simulink model "SingleTrackCANoe"  (R2021b)
settings: Solver=ode1  StartTime=0  StopTime=2  FixedStep=1.0000000000000000e-003  RelTol=1e-3
InitFcn:
  | sampleTime = str2double(get_param(bdroot, 'FixedStep'));
undefined symbols (not defined in the file or in its folder): AccPedalPos, BrakePedalPos, BrakeSwitch, DiscIntNeverNeededParam, DYNA4, EngSpd, IgnitionSwitch, InitialGear, InitialSpeed, IntendedEngTrq, LeftIndicator, MainBrakePress, MaxGear, MDL, MinGear, RefAcc, RefLane, RefLatPos, RefPath, RefPathCurv, RefSpd, RefSpdPreview, RefSpdRetrospect, RightIndicator, SteeringWheelAng, SteeringWheelTrq, UserDefinedRefValue, vm_const
libraries: UtilitiesLibrary x62, simulink x18, WheelSystemModules x14, LongitudinalControllerModules x13, LateralControllerModules x7, AnimationBusselectorModules x5, EnvironmentModules x5, BasicEngineControlModules x5, MiscellaneousControlModules x5, Animation3Modules x4, AuxiliariesModules x4, ReducedTireModules x4
(part 16 of 34)

== system SingleTrackCANoe/SimulationModel/Vehicle/WheelSystem/WheelSystemOutputs ==
  FrontLeftInnerTireStates : Inport
  FrontLeftTireStates : Inport  Port=2
  FrontLeftWheelStates : Inport  Port=3
  FrontRightInnerTireStates : Inport  Port=4
  FrontRightTireStates : Inport  Port=5
  FrontRightWheelStates : Inport  Port=6
  RearLeftInnerTireStates : Inport  Port=7
  RearLeftTireStates : Inport  Port=8
  RearLeftWheelStates : Inport  Port=9
  RearRightInnerTireStates : Inport  Port=10
  RearRightTireStates : Inport  Port=11
  RearRightWheelStates : Inport  Port=12
  FrontLeftOuput : Subsystem  Tag=TESIS DYNAware Interface Block  mask{NeedsUpdate=off, SignalInfo=|}
      mask SignalInfo=|
      | {
      |   "Version": "4.6",
      |   "MuxedOutputBusName": "FrontLeft",
      |   "MuxedInputBusName": "input",
      |   "MuxedInputSelected": false,
      |   "MuxedOutputSelected": true,
      |   "SignalData": [
      |     {
      |       "initialValue": "0.0",
      |       "name": "InnerTire",
      |       "comment": "",
      |       "minString": "",
      |       "maxString": "",
      |       "width": -1,
      |       "dataType": 0,
      |       "signalType": 1,
      |       "createSignal": false,
      |       "outputName": "InnerTire",
      |       "generateSignalAccessBlock": false,
      |       "accessId": "$(parentId).$(blockName).$(outputName)"
      |     },
      |     {
      |       "initialValue": "0.0",
      |       "name": "Tire",
      |       "comment": "",
      |       "minString": "",
      |       "maxString": "",
      |       "width": -1,
      |       "dataType": 0,
      |       "signalType": 1,
      |       "createSignal": false,
      |       "outputName": "Tire",
      |       "generateSignalAccessBlock": false,
      |       "accessId": "$(parentId).$(blockName).$(outputName)"
      |     },
      |     {
      |       "initialValue": "0.0",
      |       "name": "Wheel",
      |       "comment": "",
      |       "minString": "",
      |       "maxString": "",
      |       "width": -1,
      |       "dataType": 0,
      |       "signalType": 1,
      |       "createSignal": false,
      |       "outputName": "Wheel",
      |       "generateSignalAccessBlock": false,
      |       "accessId": "$(parentId).$(blockName).$(outputName)"
      |     }
      |   ]
      | }
      mask prompts: NeedsUpdate "Specify, if subsystem content needs to be updated"; SignalInfo "Signal Info (json)"
      mask help: DYNA4 Interface Block Version 4.6
      mask init:
      | blockName = get_param(gcbh, 'Name');
      | parentId = DYNA4.ModelHandling.AccessID.getFromHierarchy(gcbh);
      | TD.InterfaceBlock.ModelCallbacks.GenerateContent(gcb);
      settings: DeleteFcn=TD.InterfaceBlock.ModelCallbacks.CloseGUI( gcbh );  NameChangeFcn=TD.InterfaceBlock.ModelCallbacks.BlockRenamedHandler(gcbh);  OpenFcn=TD.InterfaceBlock.ModelCallbacks.OpenGUI( gcbh );  CloseFcn=TD.InterfaceBlock.ModelCallbacks.CloseGUI( gcbh );
      mask Display:
      | image('InterfaceBlock.png','center');
      | port_label('input',1, 'InnerTire');
      | port_label('input',2, 'Tire');
      | port_label('input',3, 'Wheel');
      | port_label('output',1, 'FrontLeft');
  FrontRightOuput : Subsystem  Tag=TESIS DYNAware Interface Block  mask{NeedsUpdate=off, SignalInfo=|}
      mask SignalInfo=|
      | {
      |   "Version": "4.6",
      |   "MuxedOutputBusName": "FrontRight",
      |   "MuxedInputBusName": "input",
      |   "MuxedInputSelected": false,
      |   "MuxedOutputSelected": true,
      |   "SignalData": [
      |     {
      |       "initialValue": "0.0",
      |       "name": "InnerTire",
      |       "comment": "",
      |       "minString": "",
      |       "maxString": "",
      |       "width": -1,
      |       "dataType": 0,
      |       "signalType": 1,
      |       "createSignal": false,
      |       "outputName": "InnerTire",
      |       "generateSignalAccessBlock": false,
      |       "accessId": "$(parentId).$(blockName).$(outputName)"
      |     },
      |     {
      |       "initialValue": "0.0",
      |       "name": "Tire",
      |       "comment": "",
      |       "minString": "",
      |       "maxString": "",
      |       "width": -1,
      |       "dataType": 0,
      |       "signalType": 1,
      |       "createSignal": false,
      |       "outputName": "Tire",
      |       "generateSignalAccessBlock": false,
      |       "accessId": "$(parentId).$(blockName).$(outputName)"
      |     },
      |     {
      |       "initialValue": "0.0",
      |       "name": "Wheel",
      |       "comment": "",
      |       "minString": "",
      |       "maxString": "",
      |       "width": -1,
      |       "dataType": 0,
      |       "signalType": 1,
      |       "createSignal": false,
      |       "outputName": "Wheel",
      |       "generateSignalAccessBlock": false,
      |       "accessId": "$(parentId).$(blockName).$(outputName)"
      |     }
      |   ]
      | }
      mask prompts: NeedsUpdate "Specify, if subsystem content needs to be updated"; SignalInfo "Signal Info (json)"
      mask help: DYNA4 Interface Block Version 4.6
      mask init:
      | blockName = get_param(gcbh, 'Name');
      | parentId = DYNA4.ModelHandling.AccessID.getFromHierarchy(gcbh);
      | TD.InterfaceBlock.ModelCallbacks.GenerateContent(gcb);
      settings: DeleteFcn=TD.InterfaceBlock.ModelCallbacks.CloseGUI( gcbh );  NameChangeFcn=TD.InterfaceBlock.ModelCallbacks.BlockRenamedHandler(gcbh);  OpenFcn=TD.InterfaceBlock.ModelCallbacks.OpenGUI( gcbh );  CloseFcn=TD.InterfaceBlock.ModelCallbacks.CloseGUI( gcbh );
      mask Display:
      | image('InterfaceBlock.png','center');
      | port_label('input',1, 'InnerTire');
      | port_label('input',2, 'Tire');
      | port_label('input',3, 'Wheel');
      | port_label('output',1, 'FrontRight');
  RearLeftOuput : Subsystem  Tag=TESIS DYNAware Interface Block  mask{NeedsUpdate=off, SignalInfo=|}
      mask SignalInfo=|
      | {
      |   "Version": "4.6",
      |   "MuxedOutputBusName": "RearLeft",
      |   "MuxedInputBusName": "input",
      |   "MuxedInputSelected": false,
      |   "MuxedOutputSelected": true,
      |   "SignalData": [
      |     {
      |       "initialValue": "0.0",
      |       "name": "InnerTire",
      |       "comment": "",
      |       "minString": "",
      |       "maxString": "",
      |       "width": -1,
      |       "dataType": 0,
      |       "signalType": 1,
      |       "createSignal": false,
      |       "outputName": "InnerTire",
      |       "generateSignalAccessBlock": false,
      |       "accessId": "$(parentId).$(blockName).$(outputName)"
      |     },
      |     {
      |       "initialValue": "0.0",
      |       "name": "Tire",
      |       "comment": "",
      |       "minString": "",
      |       "maxString": "",
      |       "width": -1,
      |       "dataType": 0,
      |       "signalType": 1,
      |       "createSignal": false,
      |       "outputName": "Tire",
      |       "generateSignalAccessBlock": false,
      |       "accessId": "$(parentId).$(blockName).$(outputName)"
      |     },
      |     {
      |       "initialValue": "0.0",
      |       "name": "Wheel",
      |       "comment": "",
      |       "minString": "",
      |       "maxString": "",
      |       "width": -1,
      |       "dataType": 0,
      |       "signalType": 1,
      |       "createSignal": false,
      |       "outputName": "Wheel",
      |       "generateSignalAccessBlock": false,
      |       "accessId": "$(parentId).$(blockName).$(outputName)"
      |     }
      |   ]
      | }
      mask prompts: NeedsUpdate "Specify, if subsystem content needs to be updated"; SignalInfo "Signal Info (json)"
      mask help: DYNA4 Interface Block Version 4.6
      mask init:
      | blockName = get_param(gcbh, 'Name');
      | parentId = DYNA4.ModelHandling.AccessID.getFromHierarchy(gcbh);
      | TD.InterfaceBlock.ModelCallbacks.GenerateContent(gcb);
      settings: DeleteFcn=TD.InterfaceBlock.ModelCallbacks.CloseGUI( gcbh );  NameChangeFcn=TD.InterfaceBlock.ModelCallbacks.BlockRenamedHandler(gcbh);  OpenFcn=TD.InterfaceBlock.ModelCallbacks.OpenGUI( gcbh );  CloseFcn=TD.InterfaceBlock.ModelCallbacks.CloseGUI( gcbh );
      mask Display:
      | image('InterfaceBlock.png','center');
      | port_label('input',1, 'InnerTire');
      | port_label('input',2, 'Tire');
      | port_label('input',3, 'Wheel');
      | port_label('output',1, 'RearLeft');
  RearRightOuput : Subsystem  Tag=TESIS DYNAware Interface Block  mask{NeedsUpdate=off, SignalInfo=|}
      mask SignalInfo=|
      | {
      |   "Version": "4.6",
      |   "MuxedOutputBusName": "RearRight",
      |   "MuxedInputBusName": "input",
      |   "MuxedInputSelected": false,
      |   "MuxedOutputSelected": true,
      |   "SignalData": [
      |     {
      |       "initialValue": "0.0",
      |       "name": "InnerTire",
      |       "comment": "",
      |       "minString": "",
      |       "maxString": "",
      |       "width": -1,
      |       "dataType": 0,
      |       "signalType": 1,
      |       "createSignal": false,
      |       "outputName": "InnerTire",
      |       "generateSignalAccessBlock": false,
      |       "accessId": "$(parentId).$(blockName).$(outputName)"
      |     },
      |     {
      |       "initialValue": "0.0",
      |       "name": "Tire",
      |       "comment": "",
      |       "minString": "",
      |       "maxString": "",
      |       "width": -1,
      |       "dataType": 0,
      |       "signalType": 1,
      |       "createSignal": false,
      |       "outputName": "Tire",
      |       "generateSignalAccessBlock": false,
      |       "accessId": "$(parentId).$(blockName).$(outputName)"
      |     },
      |     {
      |       "initialValue": "0.0",
      |       "name": "Wheel",
      |       "comment": "",
      |       "minString": "",
      |       "maxString": "",
      |       "width": -1,
      |       "dataType": 0,
      |       "signalType": 1,
      |       "createSignal": false,
      |       "outputName": "Wheel",
      |       "generateSignalAccessBlock": false,
      |       "accessId": "$(parentId).$(blockName).$(outputName)"
      |     }
      |   ]
      | }
      mask prompts: NeedsUpdate "Specify, if subsystem content needs to be updated"; SignalInfo "Signal Info (json)"
      mask help: DYNA4 Interface Block Version 4.6
      mask init:
      | blockName = get_param(gcbh, 'Name');
      | parentId = DYNA4.ModelHandling.AccessID.getFromHierarchy(gcbh);
      | TD.InterfaceBlock.ModelCallbacks.GenerateContent(gcb);
      settings: DeleteFcn=TD.InterfaceBlock.ModelCallbacks.CloseGUI( gcbh );  NameChangeFcn=TD.InterfaceBlock.ModelCallbacks.BlockRenamedHandler(gcbh);  OpenFcn=TD.InterfaceBlock.ModelCallbacks.OpenGUI( gcbh );  CloseFcn=TD.InterfaceBlock.ModelCallbacks.CloseGUI( gcbh );
      mask Display:
      | image('InterfaceBlock.png','center');
      | port_label('input',1, 'InnerTire');
      | port_label('input',2, 'Tire');
      | port_label('input',3, 'Wheel');
      | port_label('output',1, 'RearRight');
  WheelRear2_3Output : WheelSystemModules/WheelRear2_3Output  SystemSampleTime=-1  VariantActivationTime=update diagram  Latency=0  AutoFrameSizeCalculation=off
  WheelSystemOutput : Subsystem  Tag=TESIS DYNAware Interface Block  mask{NeedsUpdate=off, SignalInfo=|}
      mask SignalInfo=|
      | {
      |   "Version": "4.6",
      |   "MuxedOutputBusName": "WheelSystem",
      |   "MuxedInputBusName": "input",
      |   "MuxedInputSelected": false,
      |   "MuxedOutputSelected": true,
      |   "SignalData": [
      |     {
      |       "initialValue": "0.0",
      |       "name": "FrontLeft",
      |       "comment": "",
      |       "minString": "",
      |       "maxString": "",
      |       "width": -1,
      |       "dataType": 0,
      |       "signalType": 1,
      |       "createSignal": false,
      |       "outputName": "FrontLeft",
      |       "generateSignalAccessBlock": false,
      |       "accessId": "$(parentId).$(blockName).$(outputName)"
      |     },
      |     {
      |       "initialValue": "0.0",
      |       "name": "FrontRight",
      |       "comment": "",
      |       "minString": "",
      |       "maxString": "",
      |       "width": -1,
      |       "dataType": 0,
      |       "signalType": 1,
      |       "createSignal": false,
      |       "outputName": "FrontRight",
      |       "generateSignalAccessBlock": false,
      |       "accessId": "$(parentId).$(blockName).$(outputName)"
      |     },
      |     {
      |       "initialValue": "0.0",
      |       "name": "RearLeft",
      |       "comment": "",
      |       "minString": "",
      |       "maxString": "",
      |       "width": -1,
      |       "dataType": 0,
      |       "signalType": 1,
      |       "createSignal": false,
      |       "outputName": "RearLeft",
      |       "generateSignalAccessBlock": false,
      |       "accessId": "$(parentId).$(blockName).$(outputName)"
      |     },
      |     {
      |       "initialValue": "0.0",
      |       "name": "RearRight",
      |       "comment": "",
      |       "minString": "",
      |       "maxString": "",
      |       "width": -1,
      |       "dataType": 0,
      |       "signalType": 1,
      |       "createSignal": false,
      |       "outputName": "RearRight",
      |       "generateSignalAccessBlock": false,
      |       "accessId": "$(parentId).$(blockName).$(outputName)"
      |     },
      |     {
      |       "initialValue": "0.0",
      |       "name": "Rear2Left",
      |       "comment": "",
      |       "minString": "",
      |       "maxString": "",
      |       "width": -1,
      |       "dataType": 0,
      |       "signalType": 1,
      |       "createSignal": false,
      |       "outputName": "Rear2Left",
      |       "generateSignalAccessBlock": false,
      |       "accessId": "$(parentId).$(blockName).$(outputName)"
      |     },
      |     {
      |       "initialValue": "0.0",
      |       "name": "Rear2Right",
      |       "comment": "",
      |       "minString": "",
      |       "maxString": "",
      |       "width": -1,
      |       "dataType": 0,
      |       "signalType": 1,
      |       "createSignal": false,
      |       "outputName": "Rear2Right",
      |       "generateSignalAccessBlock": false,
      |       "accessId": "$(parentId).$(blockName).$(outputName)"
      |     },
      |     {
      |       "initialValue": "0.0",
      |       "name": "Rear3Left",
      |       "comment": "",
      |       "minString": "",
      |       "maxString": "",
      |       "width": -1,
      |       "dataType": 0,
      |       "signalType": 1,
      |       "createSignal": false,
      |       "outputName": "Rear3Left",
      |       "generateSignalAccessBlock": false,
      |       "accessId": "$(parentId).$(blockName).$(outputName)"
      |     },
      |     {
      |       "initialValue": "0.0",
      |       "name": "Rear3Right",
      |       "comment": "",
      |       "minString": "",
      |       "maxString": "",
      |       "width": -1,
      |       "dataType": 0,
      |       "signalType": 1,
      |       "createSignal": false,
      |       "outputName": "Rear3Right",
      |       "generateSignalAccessBlock": false,
      |       "accessId": "$(parentId).$(blockName).$(outputName)"
      |     }
      |   ]
      | }
      mask prompts: NeedsUpdate "Specify, if subsystem content needs to be updated"; SignalInfo "Signal Info (json)"
      mask help: DYNA4 Interface Block Version 4.6
      mask init:
      | blockName = get_param(gcbh, 'Name');
      | parentId = DYNA4.ModelHandling.AccessID.getFromHierarchy(gcbh);
      | TD.InterfaceBlock.ModelCallbacks.GenerateContent(gcb);
      settings: DeleteFcn=TD.InterfaceBlock.ModelCallbacks.CloseGUI( gcbh );  NameChangeFcn=TD.InterfaceBlock.ModelCallbacks.BlockRenamedHandler(gcbh);  OpenFcn=TD.InterfaceBlock.ModelCallbacks.OpenGUI( gcbh );  CloseFcn=TD.InterfaceBlock.ModelCallbacks.CloseGUI( gcbh );
      mask Display:
      | image('InterfaceBlock.png','center');
      | port_label('input',1, 'FrontLeft');
      | port_label('input',2, 'FrontRight');
      | port_label('input',3, 'RearLeft');
      | port_label('input',4, 'RearRight');
      | port_label('input',5, 'Rear2Left');
      | port_label('input',6, 'Rear2Right');
      | port_label('input',7, 'Rear3Left');
      | port_label('input',8, 'Rear3Right');
      | port_label('output',1, 'WheelSystem');
  WheelSystem : Outport  VectorParamsAs1DForOutWhenUnconnected=off
  wires:
  FrontLeftInnerTireStates/1 -> FrontLeftOuput/1(InnerTire___UNIQUE_1)
  FrontLeftTireStates/1 -> FrontLeftOuput/2(Tire___UNIQUE_1)
  FrontLeftWheelStates/1 -> FrontLeftOuput/3(Wheel___UNIQUE_1)
  RearLeftInnerTireStates/1 -> RearLeftOuput/1(InnerTire___UNIQUE_1)
  RearLeftTireStates/1 -> RearLeftOuput/2(Tire___UNIQUE_1)
  RearLeftWheelStates/1 -> RearLeftOuput/3(Wheel___UNIQUE_1)
  RearRightInnerTireStates/1 -> RearRightOuput/1(InnerTire___UNIQUE_1)
  RearRightTireStates/1 -> RearRightOuput/2(Tire___UNIQUE_1)
  RearRightWheelStates/1 -> RearRightOuput/3(Wheel___UNIQUE_1)
  FrontLeftOuput/1(FrontLeft___UNIQUE_1) -> WheelSystemOutput/1(FrontLeft___UNIQUE_1)
  FrontRightOuput/1(FrontRight___UNIQUE_1) -> WheelSystemOutput/2(FrontRight___UNIQUE_1)
  RearLeftOuput/1(RearLeft___UNIQUE_1) -> WheelSystemOutput/3(RearLeft___UNIQUE_1)
  RearRightOuput/1(RearRight___UNIQUE_1) -> WheelSystemOutput/4(RearRight___UNIQUE_1)
  WheelSystemOutput/1(WheelSystem___UNIQUE_1) -> WheelSystem/1
  FrontRightInnerTireStates/1 -> FrontRightOuput/1(InnerTire___UNIQUE_1)
  FrontRightTireStates/1 -> FrontRightOuput/2(Tire___UNIQUE_1)
  FrontRightWheelStates/1 -> FrontRightOuput/3(Wheel___UNIQUE_1)
  WheelRear2_3Output/1 -> WheelSystemOutput/5(Rear2Left___UNIQUE_1), WheelSystemOutput/6(Rear2Right___UNIQUE_1), WheelSystemOutput/7(Rear3Left___UNIQUE_1), WheelSystemOutput/8(Rear3Right___UNIQUE_1)

== system SingleTrackCANoe/SimulationModel/VehicleControl/InitialConditions/InitialConditionsOutput ==
  InitialPositionX(WorldSys)[m]___UNIQUE_1 : Inport  Description=|  PortDimensions=[1]
      | <name>InitialPositionX(WorldSys)[m]</name>
      | <comment>Initial x-position in world coordinates</comment>
  InitialPositionY(WorldSys)[m]___UNIQUE_1 : Inport  Description=|  Port=2  PortDimensions=[1]
      | <name>InitialPositionY(WorldSys)[m]</name>
      | <comment>Initial y-position in world coordinates</comment>
  InitialPositionZ(WorldSys)[m]___UNIQUE_1 : Inport  Description=|  Port=3  PortDimensions=[1]
      | <name>InitialPositionZ(WorldSys)[m]</name>
      | <comment>Initial z-position in world coordinates</comment>
  InitialRoll[rad]___UNIQUE_1 : Inport  Description=|  Port=4  PortDimensions=[1]
      | <name>InitialRoll[rad]</name>
      | <comment>Initial roll angle</comment>
  InitialPitch[rad]___UNIQUE_1 : Inport  Description=|  Port=5  PortDimensions=[1]
      | <name>InitialPitch[rad]</name>
      | <comment>Initial pitch angle</comment>
  InitialYaw[rad]___UNIQUE_1 : Inport  Description=|  Port=6  PortDimensions=[1]
      | <name>InitialYaw[rad]</name>
      | <comment>Initial yaw angle</comment>
  __TDD__InitialConditions.InitialPitch[rad] : Demux  Outputs=[1]
  __TDD__InitialConditions.InitialPositionX(WorldSys)[m] : Demux  Outputs=[1]
  __TDD__InitialConditions.InitialPositionY(WorldSys)[m] : Demux  Outputs=[1]
  __TDD__InitialConditions.InitialPositionZ(WorldSys)[m] : Demux  Outputs=[1]
  __TDD__InitialConditions.InitialRoll[rad] : Demux  Outputs=[1]
  __TDD__InitialConditions.InitialYaw[rad] : Demux  Outputs=[1]
  __TDO__InitialConditions : BusCreator  Inputs=6
  InitialConditions___UNIQUE_1 : Outport  Description=|  PortDimensions=[6]  VectorParamsAs1DForOutWhenUnconnected=off
      | <name>InitialPositionX(WorldSys)[m]</name>
      | <comment>Initial x-position in world coordinates</comment>
  wires:
  InitialPositionX(WorldSys)[m]___UNIQUE_1/1 -> __TDD__InitialConditions.InitialPositionX(WorldSys)[m]/1
  __TDD__InitialConditions.InitialPositionX(WorldSys)[m]/1 -> __TDO__InitialConditions/1  "InitialPositionX(WorldSys)[m]"
  InitialPositionY(WorldSys)[m]___UNIQUE_1/1 -> __TDD__InitialConditions.InitialPositionY(WorldSys)[m]/1
  __TDD__InitialConditions.InitialPositionY(WorldSys)[m]/1 -> __TDO__InitialConditions/2  "InitialPositionY(WorldSys)[m]"
  InitialPositionZ(WorldSys)[m]___UNIQUE_1/1 -> __TDD__InitialConditions.InitialPositionZ(WorldSys)[m]/1
  __TDD__InitialConditions.InitialPositionZ(WorldSys)[m]/1 -> __TDO__InitialConditions/3  "InitialPositionZ(WorldSys)[m]"
  InitialRoll[rad]___UNIQUE_1/1 -> __TDD__InitialConditions.InitialRoll[rad]/1
  __TDD__InitialConditions.InitialRoll[rad]/1 -> __TDO__InitialConditions/4  "InitialRoll[rad]"
  InitialPitch[rad]___UNIQUE_1/1 -> __TDD__InitialConditions.InitialPitch[rad]/1
  __TDD__InitialConditions.InitialPitch[rad]/1 -> __TDO__InitialConditions/5  "InitialPitch[rad]"
  InitialYaw[rad]___UNIQUE_1/1 -> __TDD__InitialConditions.InitialYaw[rad]/1
  __TDD__InitialConditions.InitialYaw[rad]/1 -> __TDO__InitialConditions/6  "InitialYaw[rad]"
  __TDO__InitialConditions/1 -> InitialConditions___UNIQUE_1/1  "InitialConditions"

== system SingleTrackCANoe/SimulationModel/VehicleControl/LateralControl/Disabled LateralControl ==
  SchedulerAbscissae : Inport
  CtrlSystemsAbscissae : Inport  Port=2
  PhaseTerminationVals : Inport  Port=3
  VehicleInfo : Inport  Port=4
  LatCTRL : Inport  Port=5
  ExtCtrlVariablesEnforced : Inport  Port=6
  ExtCtrlVals : Inport  Port=7
  ControlSystems : Subsystem
  ControlSystemsPreprocessor : Subsystem
  DynaSystemInfo : Subsystem  Tag=DynaSystemInfo
      mask init:
      | data = get_param(gcb, 'UserData');
      settings: OpenFcn=DYNA4.ModelHandling.System.ShowEditSystemInformationDialog(gcb);
      mask Display: disp(['Type = ', data.type, '\nName = ', data.name ])
  Terminator{,1..6} (7 alike) : Terminator
  LateralControl : Outport  VectorParamsAs1DForOutWhenUnconnected=off
  wires:
  CtrlSystemsAbscissae/1 -> Terminator6/1
  VehicleInfo/1 -> Terminator5/1
  SchedulerAbscissae/1 -> Terminator/1
  PhaseTerminationVals/1 -> Terminator1/1
  LatCTRL/1 -> Terminator4/1
  ExtCtrlVariablesEnforced/1 -> Terminator2/1
  ExtCtrlVals/1 -> Terminator3/1
  ControlSystems/1(LateralControl) -> LateralControl/1

== system SingleTrackCANoe/SimulationModel/VehicleControl/LateralControl/Enabled LateralControl ==
  SchedulerAbscissae : Inport
  CtrlSystemsAbscissae : Inport  Port=2
  PhaseTerminationVals : Inport  Port=3
  VehicleInfo : Inport  Port=4
  LatCTRL : Inport  Port=5
  ExtCtrlVariablesEnforced : Inport  Port=6
  ExtCtrlVals : Inport  Port=7
  ControlSystems : Subsystem
  ControlSystemsPreprocessor : Subsystem
  DynaSystemInfo : Subsystem  Tag=DynaSystemInfo
      mask init:
      | data = get_param(gcb, 'UserData');
      settings: OpenFcn=DYNA4.ModelHandling.System.ShowEditSystemInformationDialog(gcb);
      mask Display: disp(['Type = ', data.type, '\nName = ', data.name ])
  LateralControl : Outport  VectorParamsAs1DForOutWhenUnconnected=off
  wires:
  ControlSystems/1(LateralControl) -> LateralControl/1
  ExtCtrlVals/1 -> ControlSystemsPreprocessor/5(ExtCtrlVals)
  ExtCtrlVariablesEnforced/1 -> ControlSystemsPreprocessor/4(ExtCtrlVariablesEnforced)
  LatCTRL/1 -> ControlSystemsPreprocessor/3(LatCTRL)
  PhaseTerminationVals/1 -> ControlSystemsPreprocessor/2(PhaseTerminationVals)
  SchedulerAbscissae/1 -> ControlSystemsPreprocessor/1(SchedulerAbscissae)
  ControlSystemsPreprocessor/4(ControlInputs) -> ControlSystems/4(ControlInputs)
  ControlSystemsPreprocessor/3(SourceIdentifiers) -> ControlSystems/3(SourceIdentifiers)
  ControlSystemsPreprocessor/2(TaskIdentifiers) -> ControlSystems/2(TaskIdentifiers)
  VehicleInfo/1 -> ControlSystems/6(VehicleInfo), ControlSystemsPreprocessor/7(VehicleInfo)
  CtrlSystemsAbscissae/1 -> ControlSystems/7(CtrlSystemsAbscissae)
  ControlSystems/2(ControllerParameters) -> ControlSystemsPreprocessor/6(ControllerParameters)
  ControlSystemsPreprocessor/5(UserDefinedSignals) -> ControlSystems/5(UserDefinedSignals)
  ControlSystemsPreprocessor/1(Phase[-]) -> ControlSystems/1(Phase[-])

== system SingleTrackCANoe/SimulationModel/VehicleControl/LongitudinalControl/ControlSystems ==
  note: SpeedControl Params Module has to be located here,
      | because its PreviewTime parameter is used in other controllers, too.
  SimulationTime[s] : Inport
  Phase[-] : Inport  Port=2
  TaskIdentifiers : Inport  Port=3
  SourceIdentifiers : Inport  Port=4
  ControlInputs : Inport  Port=5
  VehicleInfoSpeedControl : Inport  Port=6
  UserDefinedSignals : Inport  Port=7
  CtrlSystemsAbscissae : Inport  Port=8
  Brake System Switch and Pedal Limitation : Subsystem
  CreateOutputBus : Subsystem
  DynaSystemInfo : Subsystem  Tag=DynaSystemInfo
      mask init:
      | data = get_param(gcb, 'UserData');
      settings: OpenFcn=DYNA4.ModelHandling.System.ShowEditSystemInformationDialog(gcb);
      mask Display: disp(['Type = ', data.type, '\nName = ', data.name ])
  Longitudinal Controller : Subsystem
  ShiftControl : LongitudinalControllerModules/ShiftControl  DATA_NODE=MDL.VehicleControl.LongitudinalControl.ControlSystems.ShiftControl  UpshiftScalingMap=MDL.VehicleControl.LongitudinalControl.ControlSystems.ShiftControl.ShiftingSpeeds.UpshiftScalingMap  DownshiftScalingMap=MDL.VehicleControl.LongitudinalControl.ControlSystems.ShiftControl.ShiftingSpeeds.DownshiftScalingMap  UpshiftOffsetMap=MDL.VehicleControl.LongitudinalControl.ControlSystems.ShiftControl.ShiftingSpeeds.UpshiftOffsetMap  DownshiftOffsetMap=MDL.VehicleControl.LongitudinalControl.ControlSystems.ShiftControl.ShiftingSpeeds.DownshiftOffsetMap  UpshiftAbsoluteSpdMap=MDL.VehicleControl.LongitudinalControl.ControlSystems.ShiftControl.ShiftingSpeeds.UpshiftAbsoluteSpdMap  DownshiftAbsoluteSpdMap=MDL.VehicleControl.LongitudinalControl.ControlSystems.ShiftControl.ShiftingSpeeds.DownshiftAbsoluteSpdMap  MinGearShiftTimeConst=MDL.VehicleControl.LongitudinalControl.ControlSystems.ShiftControl.ShiftingParameters.MinGearShiftTimeConst  NeutralToFirstGearScaling=MDL.VehicleControl.LongitudinalControl.ControlSystems.ShiftControl.ShiftingParameters.NeutralToFirstGearScaling  UpshiftAllowedWheelSlip=MDL.VehicleControl.LongitudinalControl.ControlSystems.ShiftControl.ShiftingParameters.UpshiftAllowedWheelSlip  DownshiftAllowedWheelSlip=MDL.VehicleControl.LongitudinalControl.ControlSystems.ShiftControl.ShiftingParameters.DownshiftAllowedWheelSlip  GearShiftDelayTime=MDL.VehicleControl.LongitudinalControl.ControlSystems.ShiftControl.ShiftingParameters.GearShiftDelayTime  ClutchEngageEngSpd=MDL.VehicleControl.LongitudinalControl.ControlSystems.ShiftControl.ClutchParameters.ClutchEngageEngSpd  ClutchDisengageEngSpd=MDL.VehicleControl.LongitudinalControl.ControlSystems.ShiftControl.ClutchParameters.ClutchDisengageEngSpd  ClutchDelayTime=MDL.VehicleControl.LongitudinalControl.ControlSystems.ShiftControl.ClutchParameters.ClutchDelayTime  ClutchOpenSlewRate=MDL.VehicleControl.LongitudinalControl.ControlSystems.ShiftControl.ClutchParameters.ClutchOpenSlewRate  ClutchCloseSlewRate=MDL.VehicleControl.LongitudinalControl.ControlSystems.ShiftControl.ClutchParameters.ClutchCloseSlewRate  ClutchOpeningTime=MDL.VehicleControl.LongitudinalControl.ControlSystems.ShiftControl.ClutchParameters.ClutchOpeningTime  AccPedalOpenSlewRate=MDL.VehicleControl.LongitudinalControl.ControlSystems.ShiftControl.AcceleratorPedalParameters.AccPedalOpenSlewRate  AccPedalCloseSlewRate=MDL.VehicleControl.LongitudinalControl.ControlSystems.ShiftControl.AcceleratorPedalParameters.AccPedalCloseSlewRate  ReducedAccPedalTime=MDL.VehicleControl.LongitudinalControl.ControlSystems.ShiftControl.AcceleratorPedalParameters.ReducedAccPedalTime  ReducedAccPedalPos=MDL.VehicleControl.LongitudinalControl.ControlSystems.ShiftControl.AcceleratorPedalParameters.ReducedAccPedalPos
  SpeedControl : LongitudinalControllerModules/DataContainerSpeedControl  DATA_NODE=MDL.VehicleControl.LongitudinalControl.ControlSystems.SpeedControl
  ControlOutputs : Outport  VectorParamsAs1DForOutWhenUnconnected=off
  SpeedControlParameters : Outport  Port=2  VectorParamsAs1DForOutWhenUnconnected=off
  wires:
  SpeedControl/1 -> Longitudinal Controller/5(SpeedControlParameters), SpeedControlParameters/1
  UserDefinedSignals/1 -> CreateOutputBus/4(UserDefinedSignals)
  Brake System Switch and Pedal Limitation/1(ModifiedControlOutputs) -> CreateOutputBus/1(ControlOutputs)
  CreateOutputBus/1(LongitudinalControl) -> ControlOutputs/1
  CtrlSystemsAbscissae/1 -> SpeedControl/1, Longitudinal Controller/4(CtrlSystemsAbscissae)
  ControlInputs/1 -> ShiftControl/6, Brake System Switch and Pedal Limitation/4(ControlInputs), CreateOutputBus/2(ControlInputs), Longitudinal Controller/3(ControlInputs)
  SimulationTime[s]/1 -> ShiftControl/2
  ShiftControl/1 -> Brake System Switch and Pedal Limitation/1(ControlOutputs)
  TaskIdentifiers/1 -> Brake System Switch and Pedal Limitation/2(TaskIdentifiers), ShiftControl/3, Longitudinal Controller/1("TaskIdentifiers ")
  Longitudinal Controller/1(ControlOutputs) -> ShiftControl/1
  VehicleInfoSpeedControl/1 -> Brake System Switch and Pedal Limitation/3(VehicleInfoSpeedControl), ShiftControl/5, Longitudinal Controller/6(VehicleInfoSpeedControl)
  SourceIdentifiers/1 -> SpeedControl/2, ShiftControl/4, Longitudinal Controller/2(SourceIdentifiers)
  Phase[-]/1 -> CreateOutputBus/3(Phase[-])

== system SingleTrackCANoe/SimulationModel/VehicleControl/LongitudinalControl/ControlSystemsPreprocessor ==
  SchedulerAbscissae : Inport
  PhaseTerminationVals : Inport  Port=2
  LongCTRL : Inport  Port=3
  ExtCtrlVariablesEnforced : Inport  Port=4
  ExtCtrlVals : Inport  Port=5
  VehicleInfo : Inport  Port=6
  TrafficInfo : Inport  Port=7
  CtrlSystemsAbscissae : Inport  Port=8
  SpeedControlParameters : Inport  Port=9
  Bus Selector : BusSelector  OutputSignals=PreviewTime[s]
  "External Presetting of Controller " : Subsystem
  Generation of Hold Data : Subsystem
  Generation of Speed Data : Subsystem
  Maneuver : ManeuverControlModules/LongitudinalManeuver  DATA_NODE=MDL.VehicleControl.LongitudinalControl.Maneuver  Scheduler=MDL.VehicleControl.LongitudinalControl.Maneuver.Scheduler
  ReferenceSpeedComputation : LongitudinalControllerModules/DataContainerReferenceSpeedComputation  DATA_NODE=MDL.VehicleControl.LongitudinalControl.ReferenceSpeedComputation  RoadLaneCurvatureSwitch=MDL.VehicleControl.LongitudinalControl.ReferenceSpeedComputation.RoadLaneCurvatureSwitch  MaxSpd=MDL.VehicleControl.LongitudinalControl.ReferenceSpeedComputation.MaxSpd  MaxLatAcc=MDL.VehicleControl.LongitudinalControl.ReferenceSpeedComputation.MaxLatAcc  MaxLongAcc=MDL.VehicleControl.LongitudinalControl.ReferenceSpeedComputation.MaxLongAcc  MaxLongDec=MDL.VehicleControl.LongitudinalControl.ReferenceSpeedComputation.MaxLongDec  StabilizationDistance=MDL.VehicleControl.LongitudinalControl.ReferenceSpeedComputation.StabilizationDistance  SmoothingInterval=MDL.VehicleControl.LongitudinalControl.ReferenceSpeedComputation.SmoothingInterval  UpdateInterval=MDL.VehicleControl.LongitudinalControl.ReferenceSpeedComputation.UpdateInterval  Risk=MDL.VehicleControl.LongitudinalControl.ReferenceSpeedComputation.Risk  SpeedSigns=MDL.VehicleControl.LongitudinalControl.ReferenceSpeedComputation.SpeedSigns  CollisionPrevention=MDL.VehicleControl.LongitudinalControl.ReferenceSpeedComputation.CollisionPrevention
  Switch between Data Sources : Subsystem
  Vehicle Speed Sensor : LongitudinalControllerModules/Vehicle Speed Sensor  SystemSampleTime=-1  VariantActivationTime=update diagram  Latency=0  AutoFrameSizeCalculation=off
  Phase[-] : Outport  VectorParamsAs1DForOutWhenUnconnected=off
  TaskIdentifiers : Outport  Port=2  VectorParamsAs1DForOutWhenUnconnected=off
  SourceIdentifiers : Outport  Port=3  VectorParamsAs1DForOutWhenUnconnected=off
  ControlInputs : Outport  Port=4  VectorParamsAs1DForOutWhenUnconnected=off
  VehicleInfoSpeedControl : Outport  Port=5  VectorParamsAs1DForOutWhenUnconnected=off
  UserDefinedSignals : Outport  Port=6  VectorParamsAs1DForOutWhenUnconnected=off
  wires:
  Maneuver/6 -> UserDefinedSignals/1
  Bus Selector/1 -> Maneuver/3, Generation of Speed Data/7(PreviewTime[s])  "<PreviewTime[s]>"
  ReferenceSpeedComputation/1 -> Generation of Speed Data/4(ReferenceSpeedParameters)
  CtrlSystemsAbscissae/1 -> ReferenceSpeedComputation/1
  TrafficInfo/1 -> Generation of Speed Data/6(TrafficInfo)
  ExtCtrlVariablesEnforced/1 -> "External Presetting of Controller "/3(ExtCtrlVariablesEnforced)
  "External Presetting of Controller "/1(ModifiedTaskIdentifiers) -> TaskIdentifiers/1, Generation of Speed Data/1(TaskIdentifiers)
  LongCTRL/1 -> Generation of Hold Data/2(LongCTRL)
  Generation of Hold Data/1(HoldData) -> Switch between Data Sources/3(HoldData)
  Switch between Data Sources/1(SwitchedControlInputs) -> Generation of Speed Data/3(ControlInputs)
  Generation of Speed Data/1(ModifiedControlInputs) -> ControlInputs/1
  Maneuver/3 -> "External Presetting of Controller "/1(TaskIdentifiers)
  SchedulerAbscissae/1 -> Maneuver/1
  PhaseTerminationVals/1 -> Maneuver/2
  Maneuver/4 -> "External Presetting of Controller "/2(SourceIdentifiers)
  Maneuver/2 -> Generation of Hold Data/1(PhaseTrigger)
  "External Presetting of Controller "/2(ModifiedSourceIdentifiers) -> Switch between Data Sources/1(SourceIdentifiers), Generation of Speed Data/2(SourceIdentifiers), SourceIdentifiers/1
  SpeedControlParameters/1 -> Bus Selector/1, Vehicle Speed Sensor/1
  ExtCtrlVals/1 -> Switch between Data Sources/4(ExternalData)
  Maneuver/5 -> Generation of Hold Data/4(ControlInputs), Switch between Data Sources/2(ControlInputs)
  Maneuver/1 -> Phase[-]/1
  Vehicle Speed Sensor/1 -> Generation of Hold Data/3(VehicleInfo), VehicleInfoSpeedControl/1, Generation of Speed Data/5(VehicleInfo)
  VehicleInfo/1 -> Vehicle Speed Sensor/2

== system SingleTrackCANoe/SimulationModel/VehicleControl/LongitudinalControl/DynaSystemInfo ==

== system SingleTrackCANoe/SimulationModel/VehicleControl/Miscellaneous/DynaSystemInfo ==

== system SingleTrackCANoe/SimulationModel/VehicleControl/Miscellaneous/UserDefinedControlOutput ==
  UserDefined1[-]___UNIQUE_1 : Inport  Description=|  PortDimensions=[1]
      | <name>UserDefined1[-]</name>
      | <comment>User-defined miscellaneous signal 1 (can be edited by the user) </comment>
  UserDefined2[-]___UNIQUE_1 : Inport  Description=|  Port=2  PortDimensions=[1]
      | <name>UserDefined2[-]</name>
      | <comment>User-defined miscellaneous signal 2 (can be edited by the user) </comment>
  __TDD__UserDefinedControl.UserDefined1[-] : Demux  Outputs=[1]
  __TDD__UserDefinedControl.UserDefined2[-] : Demux  Outputs=[1]
  __TDO__UserDefinedControl : BusCreator  Inputs=2
  UserDefinedControl___UNIQUE_1 : Outport  Description=|  PortDimensions=[2]  VectorParamsAs1DForOutWhenUnconnected=off
      | <name>UserDefined1[-]</name>
      | <comment>User-defined miscellaneous signal 1 (can be edited by the user) </comment>
  wires:
  UserDefined1[-]___UNIQUE_1/1 -> __TDD__UserDefinedControl.UserDefined1[-]/1
  __TDD__UserDefinedControl.UserDefined1[-]/1 -> __TDO__UserDefinedControl/1  "UserDefined1[-]"
  UserDefined2[-]___UNIQUE_1/1 -> __TDD__UserDefinedControl.UserDefined2[-]/1
  __TDD__UserDefinedControl.UserDefined2[-]/1 -> __TDO__UserDefinedControl/2  "UserDefined2[-]"
  __TDO__UserDefinedControl/1 -> UserDefinedControl___UNIQUE_1/1  "UserDefinedControl"

== system SingleTrackCANoe/SimulationModel/VehicleControl/VehicleControlInputs/CreateLatExtCtrlDataBus ==
  FromCTRL : Inport
  Bus Assignment : BusAssignment  AssignedSignals=RefLatPos,RefLane,RefPath,RefPathCurv,UserDefinedRefValue
  Bus Selector : BusSelector  OutputSignals=CTRL_LateralControl_RefLatPos[m],CTRL_LateralControl_RefLane[-],CTRL_LateralControl_RefPath[-],CTRL_LateralControl_RefCurv[1/m],CTRL_LateralControl_UserDefinedRefValue[-]
  TD_BO_LateralControlInputs all zero : Constant  Value=0  OutDataTypeStr=Bus: TD_BO_LateralControlInputs
  needed due to bus unit comparisons : Gain
  needed due to bus unit comparisons1 : Gain
  DataBus : Outport  OutDataTypeStr=Bus: TD_BO_LateralControlInputs  VectorParamsAs1DForOutWhenUnconnected=off
  wires:
  needed due to bus unit comparisons1/1 -> Bus Assignment/5
  needed due to bus unit comparisons/1 -> Bus Assignment/2
  TD_BO_LateralControlInputs all zero/1 -> Bus Assignment/1
  Bus Selector/2 -> Bus Assignment/3  "<CTRL_LateralControl_RefLane[-]>"
  Bus Selector/1 -> needed due to bus unit comparisons/1  "<CTRL_LateralControl_RefLatPos[m]>"
  Bus Selector/4 -> needed due to bus unit comparisons1/1  "<CTRL_LateralControl_RefCurv[1/m]>"
  Bus Selector/3 -> Bus Assignment/4  "<CTRL_LateralControl_RefPath[-]>"
  Bus Selector/5 -> Bus Assignment/6  "<CTRL_LateralControl_UserDefinedRefValue[-]>"
  Bus Assignment/1 -> DataBus/1
  FromCTRL/1 -> Bus Selector/1

== system SingleTrackCANoe/SimulationModel/VehicleControl/VehicleControlInputs/CreateLongExtCtrlDataBus ==
  FromCTRL : Inport
  All zeros TD_BO_LongitudinalControlInputs : Constant  Value=0  OutDataTypeStr=Bus: TD_BO_LongitudinalControlInputs
  Bus Assignment : BusAssignment  AssignedSignals=RefSpd,RefSpdPreview,RefSpdRetrospect,RefAcc,UserDefinedRefValue
  Bus Selector : BusSelector  OutputSignals=CTRL_LongitudinalControl_RefSpd[m/s],CTRL_LongitudinalControl_RefAcc[m/s**2],CTRL_LongitudinalControl_UserDefinedRefValue[-]
  needed due to bus unit comparisons : Gain
  needed due to bus unit comparisons1 : Gain
  DataBus : Outport  VectorParamsAs1DForOutWhenUnconnected=off
  wires:
  needed due to bus unit comparisons1/1 -> Bus Assignment/5
  needed due to bus unit comparisons/1 -> Bus Assignment/3, Bus Assignment/2, Bus Assignment/4
  All zeros TD_BO_LongitudinalControlInputs/1 -> Bus Assignment/1
  Bus Assignment/1 -> DataBus/1
  Bus Selector/1 -> needed due to bus unit comparisons/1  "<CTRL_LongitudinalControl_RefSpd[m/s]>"
  Bus Selector/2 -> needed due to bus unit comparisons1/1  "<CTRL_LongitudinalControl_RefAcc[m/s**2]>"
  Bus Selector/3 -> Bus Assignment/6  "<CTRL_LongitudinalControl_UserDefinedRefValue[-]>"
  FromCTRL/1 -> Bus Selector/1
